simulink model "untitled1"  (R2019b)
settings: Solver=VariableStepAuto  StartTime=0.0  StopTime=5  RelTol=1e-3
values from neighbouring files (symbols this model uses):
  Brad = 0.17    [lab6.m]    (also in multiple_V.m)
  J = 0.0023    [lab6.m]    (also in multiple_V.m)
  Ke = Km    (= 0.29)    [lab6.m]    (also in multiple_V.m)
  Km = 0.29    [lab6.m]    (also in multiple_V.m)
  Kr = 100    [lab6.m]    (also in multiple_V.m)
  L = 0.0047    [lab6.m]    (also in multiple_V.m)
  R = 4.7    [lab6.m]    (also in multiple_V.m)
  Rad = 0.0275    [lab6.m]    (also in multiple_V.m)
  Um = 3.5    [lab6.m]    (also in multiple_V.m)
settings Model: Creator=Ivan  LastModifiedBy=Ivan

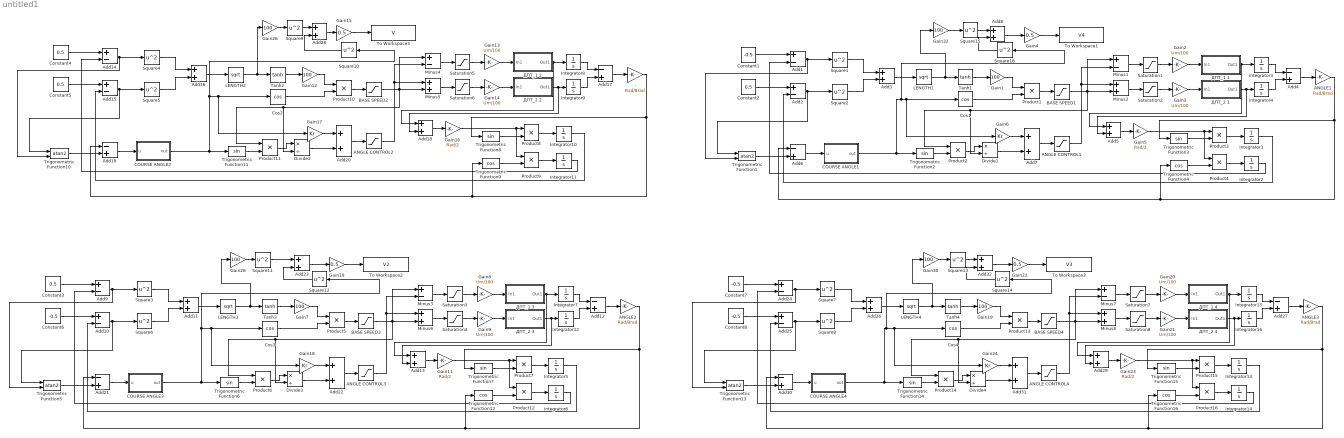
== system untitled1 ==
  - : Gain  Gain=Rad/Brad
  ANGLE CONTROL{1..4} (4 alike) : Saturate  UpperLimit=20  LowerLimit=-20
  ANGLE1 : Gain  Gain=Rad/Brad
  ANGLE2 : Gain  Gain=Rad/Brad
  ANGLE3 : Gain  Gain=Rad/Brad
  Add{1..2,9..10,14..15,24..25} (8 alike) : Sum  Inputs=+-
  Add{3,5,7..8,11,13,16,18,20,22..23,26,28..29,31..32} (16 alike) : Sum
  Add{4,6,12,17,19,21,27,30} (8 alike) : Sum  Inputs=-+
  BASE SPEED{1..4} (4 alike) : Saturate  UpperLimit=80  LowerLimit=-80
  COURSE ANGLE1 : MATLAB Function  TreatAsAtomicUnit=on  VariantControl=Variant1
  COURSE ANGLE2 : MATLAB Function  TreatAsAtomicUnit=on  VariantControl=Variant1
  COURSE ANGLE3 : MATLAB Function  TreatAsAtomicUnit=on  VariantControl=Variant1
  COURSE ANGLE4 : MATLAB Function  TreatAsAtomicUnit=on  VariantControl=Variant1
  Constant{1,6..8} (4 alike) : Constant  Value=-0.5
  Constant{2..5} (4 alike) : Constant  Value=0.5
  Cos{1..4} (4 alike) : Trigonometry  Operator=cos
  Divide{1..4} (4 alike) : Product  Inputs=*/
  Gain{1,7,12,19,26,28,30,32} (8 alike) : Gain  Gain=100
  Gain{4,10,15,22} (4 alike) : Gain  Gain=0.5
  Gain{5,11,16,23} (4 alike) : Gain  Gain=Rad/2
  Gain{2..3,8..9,13..14,20..21} (8 alike) : Gain  Gain=Um/100
  Gain{6,17..18,24} (4 alike) : Gain  Gain=Kr
  Integrator{1..16} (16 alike) : Integrator
  LENGTH{1..4} (4 alike) : Sqrt  SaturateOnIntegerOverflow=on
  Minus{1,3..4,7} (4 alike) : Sum  Inputs=+-
  Minus{2,5..6,8} (4 alike) : Sum
  Product{1..16} (16 alike) : Product
  Saturation{1..8} (8 alike) : Saturate  UpperLimit=100  LowerLimit=-100
  Square{1..16} (16 alike) : Math  Operator=square  SignedPower=off  SaturateOnIntegerOverflow=on
  Tanh{1..4} (4 alike) : Trigonometry  Operator=tanh
  To Workspace1 : ToWorkspace  VariableName=V4  SaveFormat=Timeseries  SampleTime=-1
  To Workspace2 : ToWorkspace  VariableName=V2  SaveFormat=Timeseries  SampleTime=-1
  To Workspace3 : ToWorkspace  VariableName=V3  SaveFormat=Timeseries  SampleTime=-1
  To Workspace5 : ToWorkspace  VariableName=V  SaveFormat=Timeseries  SampleTime=-1
  Trigonometric Function{1,5,10,13} (4 alike) : Trigonometry  Operator=atan2
  Trigonometric Function{2..3,6..8,11,14..15} (8 alike) : Trigonometry
  Trigonometric Function{4,9,12,16} (4 alike) : Trigonometry  Operator=cos
  ДПТ_1 1 : Subsystem
  ДПТ_1 2 : Subsystem
  ДПТ_1 3 : Subsystem
  ДПТ_1 4 : Subsystem
  ДПТ_2 1 : Subsystem
  ДПТ_2 2 : Subsystem
  ДПТ_2 3 : Subsystem
  ДПТ_2 4 : Subsystem
  wires:
  Constant4/1 -> Add14/1
  Constant5/1 -> Add15/1
  Tanh2/1 -> Gain12/1
  Add19/1 -> COURSE ANGLE2/1(u)
  Saturation6/1 -> Gain14/1
  Integrator11/1 -> Add14/2
  -/1 -> Trigonometric Function8/1, Trigonometric Function9/1, Add19/1
  ANGLE CONTROL2/1 -> Minus4/2, Minus5/1
  Add20/1 -> ANGLE CONTROL2/1
  Product9/1 -> Integrator11/1
  Product11/1 -> Divide2/1
  ДПТ_2 2/1(Out1) -> Add18/2, Integrator9/1
  Divide2/1 -> Add20/2
  Minus4/1 -> Saturation5/1
  Minus5/1 -> Saturation6/1
  Trigonometric Function10/1 -> Add19/2
  Add18/1 -> Gain16/1
  Add17/1 -> -/1
  Gain13/1 -> ДПТ_1 2/1(In1)
  Square4/1 -> Add16/1
  Integrator9/1 -> Add17/2
  Add16/1 -> LENGTH2/1
  Trigonometric Function8/1 -> Product8/2
  Gain17/1 -> Add20/1
  Saturation5/1 -> Gain13/1
  Integrator8/1 -> Add17/1
  Add14/1 -> Trigonometric Function10/2, Square4/1
  Product8/1 -> Integrator10/1
  Product10/1 -> BASE SPEED2/1
  ДПТ_1 2/1(Out1) -> Add18/1, Integrator8/1
  Cos2/1 -> Product10/2
  Gain12/1 -> Product10/1
  Add15/1 -> Trigonometric Function10/1, Square5/1
  LENGTH2/1 -> Gain26/1, Tanh2/1
  Square5/1 -> Add16/2
  BASE SPEED2/1 -> Minus4/1, Minus5/2, Divide2/2, Product11/1
  Trigonometric Function9/1 -> Product9/2
  Integrator10/1 -> Add15/2
  Gain16/1 -> Product9/1, Product8/1
  Trigonometric Function11/1 -> Product11/2
  Gain14/1 -> ДПТ_2 2/1(In1)
  Add28/1 -> Gain15/1
  Gain15/1 -> To Workspace5/1
  Add5/1 -> Gain5/1
  Add4/1 -> ANGLE1/1
  Trigonometric Function1/1 -> Add6/2
  Integrator4/1 -> Add4/2
  Gain2/1 -> ДПТ_1 1/1(In1)
  Square1/1 -> Add3/1
  Minus2/1 -> Saturation2/1
  Minus1/1 -> Saturation1/1
  Divide1/1 -> Add7/2
  Product2/1 -> Divide1/1
  ANGLE1/1 -> Trigonometric Function3/1, Trigonometric Function4/1, Add6/1
  ДПТ_2 1/1(Out1) -> Add5/2, Integrator4/1
  Integrator2/1 -> Add1/2
  Trigonometric Function2/1 -> Product2/2
  Gain3/1 -> ДПТ_2 1/1(In1)
  Saturation2/1 -> Gain3/1
  Product4/1 -> Integrator2/1
  Constant2/1 -> Add2/1
  Tanh1/1 -> Gain1/1
  Square2/1 -> Add3/2
  Constant1/1 -> Add1/1
  Add7/1 -> ANGLE CONTROL1/1
  Add2/1 -> Trigonometric Function1/1, Square2/1
  Cos1/1 -> Product1/2
  LENGTH1/1 -> Gain32/1, Tanh1/1
  Product3/1 -> Integrator1/1
  Product1/1 -> BASE SPEED1/1
  Integrator3/1 -> Add4/1
  Saturation1/1 -> Gain2/1
  Gain6/1 -> Add7/1
  Add6/1 -> COURSE ANGLE1/1(u)
  Add3/1 -> LENGTH1/1
  Add1/1 -> Trigonometric Function1/2, Square1/1
  Gain1/1 -> Product1/1
  Trigonometric Function3/1 -> Product3/2
  BASE SPEED1/1 -> Minus1/1, Minus2/2, Divide1/2, Product2/1
  Trigonometric Function4/1 -> Product4/2
  Gain5/1 -> Product4/1, Product3/1
  Integrator1/1 -> Add2/2
  Gain4/1 -> To Workspace1/1
  Add8/1 -> Gain4/1
  ДПТ_1 1/1(Out1) -> Add5/1, Integrator3/1
  ANGLE CONTROL1/1 -> Minus1/2, Minus2/1
  Add13/1 -> Gain11/1
  Add12/1 -> ANGLE2/1
  Trigonometric Function5/1 -> Add21/2
  Integrator12/1 -> Add12/2
  Gain8/1 -> ДПТ_1 3/1(In1)
  Square3/1 -> Add11/1
  Minus6/1 -> Saturation4/1
  Minus3/1 -> Saturation3/1
  Divide3/1 -> Add22/2
  Product6/1 -> Divide3/1
  ANGLE2/1 -> Trigonometric Function7/1, Trigonometric Function12/1, Add21/1
  ДПТ_2 3/1(Out1) -> Add13/2, Integrator12/1
  Integrator6/1 -> Add9/2
  Trigonometric Function6/1 -> Product6/2
  Gain9/1 -> ДПТ_2 3/1(In1)
  Saturation4/1 -> Gain9/1
  Product12/1 -> Integrator6/1
  Constant6/1 -> Add10/1
  Tanh3/1 -> Gain7/1
  Square6/1 -> Add11/2
  Constant3/1 -> Add9/1
  Add22/1 -> ANGLE CONTROL3/1
  Add10/1 -> Trigonometric Function5/1, Square6/1
  Cos3/1 -> Product5/2
  LENGTH3/1 -> Gain28/1, Tanh3/1
  Product7/1 -> Integrator5/1
  Product5/1 -> BASE SPEED3/1
  Integrator7/1 -> Add12/1
  Saturation3/1 -> Gain8/1
  Gain18/1 -> Add22/1
  Add21/1 -> COURSE ANGLE3/1(u)
  Add11/1 -> LENGTH3/1
  Add9/1 -> Trigonometric Function5/2, Square3/1
  Gain7/1 -> Product5/1
  Trigonometric Function7/1 -> Product7/2
  BASE SPEED3/1 -> Minus3/1, Minus6/2, Divide3/2, Product6/1
  Trigonometric Function12/1 -> Product12/2
  Gain11/1 -> Product12/1, Product7/1
  Integrator5/1 -> Add10/2
  Gain10/1 -> To Workspace2/1
  Add23/1 -> Gain10/1
  ДПТ_1 3/1(Out1) -> Add13/1, Integrator7/1
  ANGLE CONTROL3/1 -> Minus3/2, Minus6/1
  Add29/1 -> Gain23/1
  Add27/1 -> ANGLE3/1
  Trigonometric Function13/1 -> Add30/2
  Integrator16/1 -> Add27/2
  Gain20/1 -> ДПТ_1 4/1(In1)
  Square7/1 -> Add26/1
  Minus8/1 -> Saturation8/1
  Minus7/1 -> Saturation7/1
  Divide4/1 -> Add31/2
  Product14/1 -> Divide4/1
  ANGLE3/1 -> Trigonometric Function15/1, Trigonometric Function16/1, Add30/1
  ДПТ_2 4/1(Out1) -> Add29/2, Integrator16/1
  Integrator14/1 -> Add24/2
  Trigonometric Function14/1 -> Product14/2
  Gain21/1 -> ДПТ_2 4/1(In1)
  Saturation8/1 -> Gain21/1
  Product16/1 -> Integrator14/1
  Constant8/1 -> Add25/1
  Tanh4/1 -> Gain19/1
  Square8/1 -> Add26/2
  Constant7/1 -> Add24/1
  Add31/1 -> ANGLE CONTROL4/1
  Add25/1 -> Trigonometric Function13/1, Square8/1
  Cos4/1 -> Product13/2
  LENGTH4/1 -> Gain30/1, Tanh4/1
  Product15/1 -> Integrator13/1
  Product13/1 -> BASE SPEED4/1
  Integrator15/1 -> Add27/1
  Saturation7/1 -> Gain20/1
  Gain24/1 -> Add31/1
  Add30/1 -> COURSE ANGLE4/1(u)
  Add26/1 -> LENGTH4/1
  Add24/1 -> Trigonometric Function13/2, Square7/1
  Gain19/1 -> Product13/1
  Trigonometric Function15/1 -> Product15/2
  BASE SPEED4/1 -> Minus7/1, Minus8/2, Divide4/2, Product14/1
  Trigonometric Function16/1 -> Product16/2
  Gain23/1 -> Product16/1, Product15/1
  Integrator13/1 -> Add25/2
  Gain22/1 -> To Workspace3/1
  Add32/1 -> Gain22/1
  ДПТ_1 4/1(Out1) -> Add29/1, Integrator15/1
  ANGLE CONTROL4/1 -> Minus7/2, Minus8/1
  COURSE ANGLE2/1(out) -> Trigonometric Function11/1, Square10/1, Gain17/1, Cos2/1
  Gain26/1 -> Square9/1
  Gain28/1 -> Square11/1
  COURSE ANGLE3/1(out) -> Trigonometric Function6/1, Square12/1, Gain18/1, Cos3/1
  Gain30/1 -> Square13/1
  COURSE ANGLE4/1(out) -> Trigonometric Function14/1, Square14/1, Gain24/1, Cos4/1
  Gain32/1 -> Square15/1
  COURSE ANGLE1/1(out) -> Trigonometric Function2/1, Square16/1, Gain6/1, Cos1/1
  Square9/1 -> Add28/1
  Square10/1 -> Add28/2
  Square11/1 -> Add23/1
  Square12/1 -> Add23/2
  Square13/1 -> Add32/1
  Square14/1 -> Add32/2
  Square15/1 -> Add8/1
  Square16/1 -> Add8/2

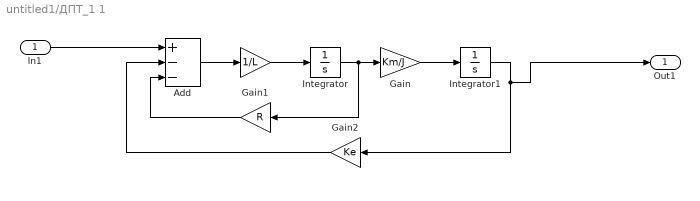
== system untitled1/ДПТ_1 1 ==
  In1 : Inport
  " " : Gain  Gain=1/L
  Add : Sum  Inputs=+--
  Gain : Gain  Gain=Km/J
  Gain1 : Gain  Gain=R
  Gain2 : Gain  Gain=Ke
  Integrator : Integrator
  Integrator1 : Integrator
  Out1 : Outport
  wires:
  In1/1 -> Add/1
  Add/1 -> " "/1
  " "/1 -> Integrator/1
  Integrator/1 -> Gain1/1, Gain/1
  Gain/1 -> Integrator1/1
  Integrator1/1 -> Out1/1, Gain2/1
  Gain1/1 -> Add/3
  Gain2/1 -> Add/2

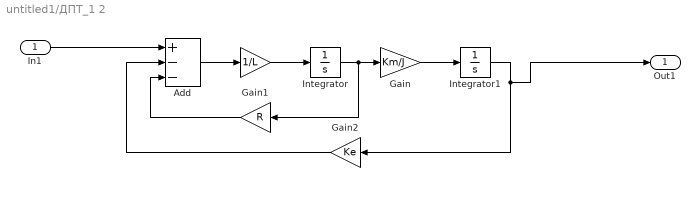
== system untitled1/ДПТ_1 2 ==
  In1 : Inport
  " " : Gain  Gain=1/L
  Add : Sum  Inputs=+--
  Gain : Gain  Gain=Km/J
  Gain1 : Gain  Gain=R
  Gain2 : Gain  Gain=Ke
  Integrator : Integrator
  Integrator1 : Integrator
  Out1 : Outport
  wires:
  In1/1 -> Add/1
  Add/1 -> " "/1
  " "/1 -> Integrator/1
  Integrator/1 -> Gain1/1, Gain/1
  Gain/1 -> Integrator1/1
  Integrator1/1 -> Out1/1, Gain2/1
  Gain1/1 -> Add/3
  Gain2/1 -> Add/2

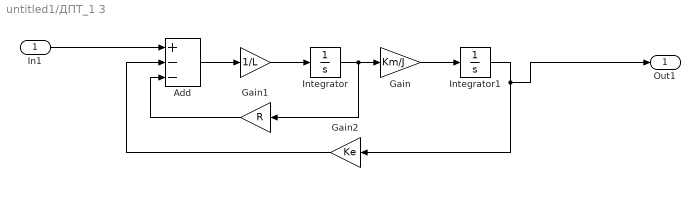
== system untitled1/ДПТ_1 3 ==
  In1 : Inport
  " " : Gain  Gain=1/L
  Add : Sum  Inputs=+--
  Gain : Gain  Gain=Km/J
  Gain1 : Gain  Gain=R
  Gain2 : Gain  Gain=Ke
  Integrator : Integrator
  Integrator1 : Integrator
  Out1 : Outport
  wires:
  In1/1 -> Add/1
  Add/1 -> " "/1
  " "/1 -> Integrator/1
  Integrator/1 -> Gain1/1, Gain/1
  Gain/1 -> Integrator1/1
  Integrator1/1 -> Out1/1, Gain2/1
  Gain1/1 -> Add/3
  Gain2/1 -> Add/2

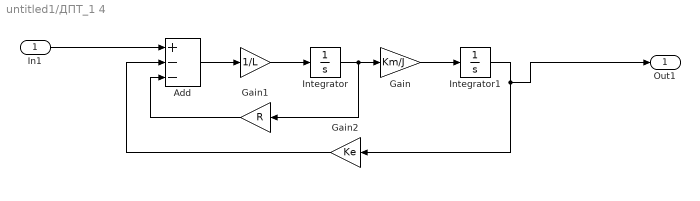
== system untitled1/ДПТ_1 4 ==
  In1 : Inport
  " " : Gain  Gain=1/L
  Add : Sum  Inputs=+--
  Gain : Gain  Gain=Km/J
  Gain1 : Gain  Gain=R
  Gain2 : Gain  Gain=Ke
  Integrator : Integrator
  Integrator1 : Integrator
  Out1 : Outport
  wires:
  In1/1 -> Add/1
  Add/1 -> " "/1
  " "/1 -> Integrator/1
  Integrator/1 -> Gain1/1, Gain/1
  Gain/1 -> Integrator1/1
  Integrator1/1 -> Out1/1, Gain2/1
  Gain1/1 -> Add/3
  Gain2/1 -> Add/2

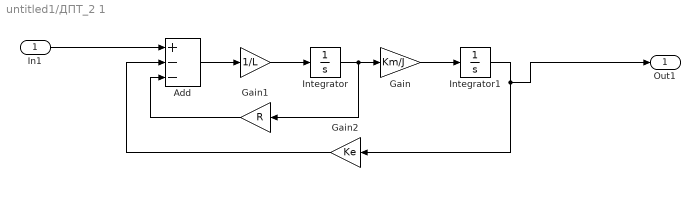
== system untitled1/ДПТ_2 1 ==
  In1 : Inport
  " " : Gain  Gain=1/L
  Add : Sum  Inputs=+--
  Gain : Gain  Gain=Km/J
  Gain1 : Gain  Gain=R
  Gain2 : Gain  Gain=Ke
  Integrator : Integrator
  Integrator1 : Integrator
  Out1 : Outport
  wires:
  In1/1 -> Add/1
  Add/1 -> " "/1
  " "/1 -> Integrator/1
  Integrator/1 -> Gain1/1, Gain/1
  Gain/1 -> Integrator1/1
  Integrator1/1 -> Out1/1, Gain2/1
  Gain1/1 -> Add/3
  Gain2/1 -> Add/2

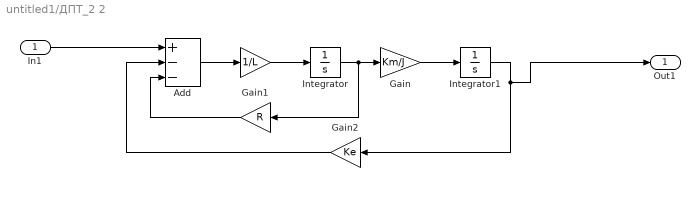
== system untitled1/ДПТ_2 2 ==
  In1 : Inport
  " " : Gain  Gain=1/L
  Add : Sum  Inputs=+--
  Gain : Gain  Gain=Km/J
  Gain1 : Gain  Gain=R
  Gain2 : Gain  Gain=Ke
  Integrator : Integrator
  Integrator1 : Integrator
  Out1 : Outport
  wires:
  In1/1 -> Add/1
  Add/1 -> " "/1
  " "/1 -> Integrator/1
  Integrator/1 -> Gain1/1, Gain/1
  Gain/1 -> Integrator1/1
  Integrator1/1 -> Out1/1, Gain2/1
  Gain1/1 -> Add/3
  Gain2/1 -> Add/2

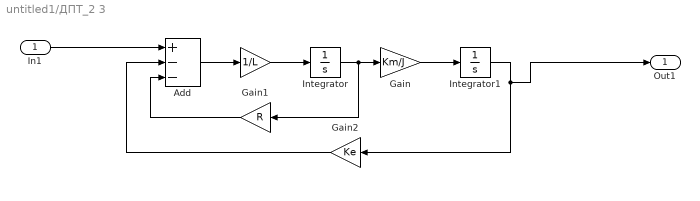
== system untitled1/ДПТ_2 3 ==
  In1 : Inport
  " " : Gain  Gain=1/L
  Add : Sum  Inputs=+--
  Gain : Gain  Gain=Km/J
  Gain1 : Gain  Gain=R
  Gain2 : Gain  Gain=Ke
  Integrator : Integrator
  Integrator1 : Integrator
  Out1 : Outport
  wires:
  In1/1 -> Add/1
  Add/1 -> " "/1
  " "/1 -> Integrator/1
  Integrator/1 -> Gain1/1, Gain/1
  Gain/1 -> Integrator1/1
  Integrator1/1 -> Out1/1, Gain2/1
  Gain1/1 -> Add/3
  Gain2/1 -> Add/2

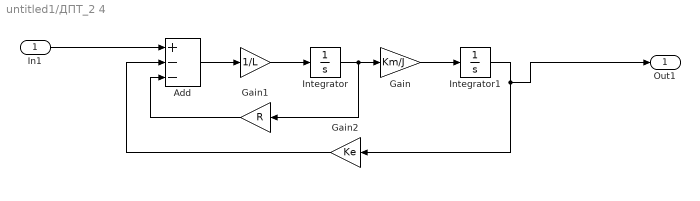
== system untitled1/ДПТ_2 4 ==
  In1 : Inport
  " " : Gain  Gain=1/L
  Add : Sum  Inputs=+--
  Gain : Gain  Gain=Km/J
  Gain1 : Gain  Gain=R
  Gain2 : Gain  Gain=Ke
  Integrator : Integrator
  Integrator1 : Integrator
  Out1 : Outport
  wires:
  In1/1 -> Add/1
  Add/1 -> " "/1
  " "/1 -> Integrator/1
  Integrator/1 -> Gain1/1, Gain/1
  Gain/1 -> Integrator1/1
  Integrator1/1 -> Out1/1, Gain2/1
  Gain1/1 -> Add/3
  Gain2/1 -> Add/2

== matlab function untitled1/COURSE ANGLE1 ==
  data: u input; out output
function out = fcn(u)
%%codegen
    if (abs(u)>3.14)
        y=u-sign(u)*2*3.14;
    else
        y=u;
    end
out = y;

== matlab function untitled1/COURSE ANGLE3 ==
  data: u input; out output
function out = fcn(u)
%%codegen
    if (abs(u)>3.14)
        y=u-sign(u)*2*3.14;
    else
        y=u;
    end
out = y;

== matlab function untitled1/COURSE ANGLE2 ==
  data: u input; out output
function out = fcn(u)
%%codegen
    if (abs(u)>3.14)
        y=u-sign(u)*2*3.14;
    else
        y=u;
    end
out = y;

== matlab function untitled1/COURSE ANGLE4 ==
  data: u input; out output
function out = fcn(u)
%%codegen
    if (abs(u)>3.14)
        y=u-sign(u)*2*3.14;
    else
        y=u;
    end
out = y;
